simulink model "openloopresponse"  (R2018a)
settings: Solver=VariableStepAuto  StartTime=0.0  StopTime=130  RelTol=1e-3
values from neighbouring files (symbols this model uses):
  KT = 0.25    [DC_Motormfile.m]    (also in pid.m)
  L = 493*10^-9    (= 4.93e-07)    [DC_Motormfile.m]    (also in pid.m)
  R = 5.3*10^-3    (= 0.0053)    [DC_Motormfile.m]    (also in pid.m)
  Ts = 0.01    [pid.m]
libraries: simulink x2
settings Model: Creator=MAFAZ  LastModifiedBy=MAFAZ

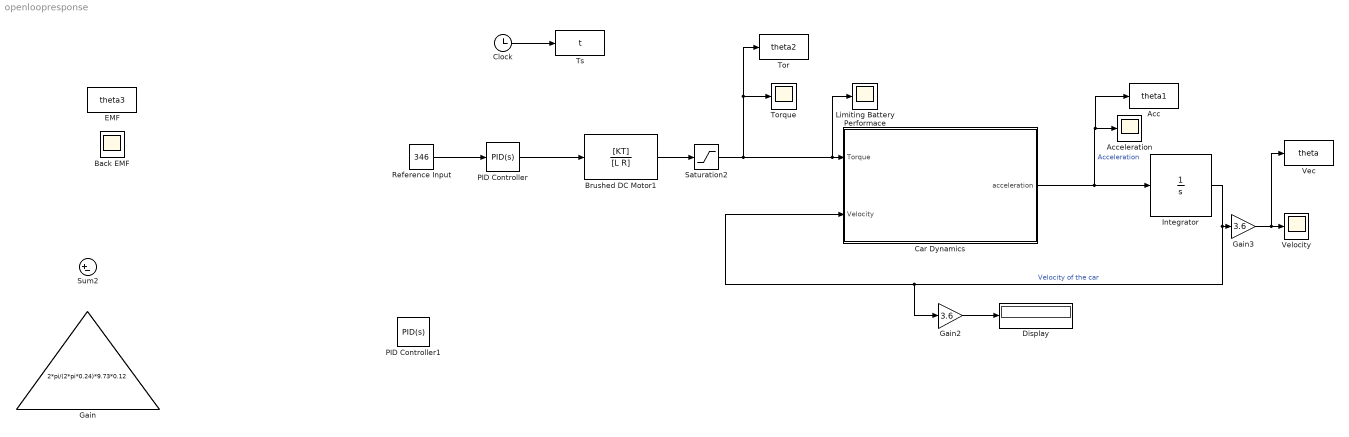
== system openloopresponse ==
  Acc : ToWorkspace  VariableName=theta1  SampleTime=Ts
  Acceleration : Scope
  Back EMF : Scope
  Brushed DC Motor1 : TransferFcn  Numerator=[KT]  Denominator=[L R]
  Car Dynamics : MATLAB Function  TreatAsAtomicUnit=on
  Clock : Clock
  Display : Display
  EMF : ToWorkspace  VariableName=theta3  SampleTime=Ts
  Gain : Gain  Gain=2*pi/(2*pi*0.24)*9.73*0.12
  Gain2 : Gain  Gain=3.6
  Gain3 : Gain  Gain=3.6
  Integrator : Integrator
  "Limiting Battery Performace " : Scope
  PID Controller : simulink/Continuous/PID Controller  Controller=PID  TimeDomain=Continuous-time  SampleTime=-1  IntegratorMethod=Forward Euler  FilterMethod=Forward Euler  Form=Parallel  UseFilter=on  ControllerParametersSource=internal  P=1000  I=500  D=0  N=100  InitialConditionSource=internal  InitialConditionForIntegrator=0  InitialConditionForFilter=0  ExternalReset=none  LimitOutput=on  UpperSaturationLimit=346  LowerSaturationLimit=0  LinearizeAsGain=on  AntiWindupMode=none  Kb=1  TrackingMode=off  Kt=1  PParamMin=[]  PParamMax=[]  IParamMin=[]  IParamMax=[]  DParamMin=[]  DParamMax=[]  NParamMin=[]  NParamMax=[]  KbParamMin=[]  KbParamMax=[]  KtParamMin=[]  KtParamMax=[]  POutMin=[]  POutMax=[]  IOutMin=[]  IOutMax=[]  DOutMin=[]  DOutMax=[]  NOutMin=[]  NOutMax=[]  KbOutMin=[]  KbOutMax=[]  KtOutMin=[]  KtOutMax=[]  IntegratorOutMin=[]  IntegratorOutMax=[]  FilterOutMin=[]  FilterOutMax=[]  SumOutMin=[]  SumOutMax=[]  SumI1OutMin=[]  SumI1OutMax=[]  SumI2OutMin=[]  SumI2OutMax=[]  SumI3OutMin=[]  SumI3OutMax=[]  SumDOutMin=[]  SumDOutMax=[]  SaturationOutMin=[]  SaturationOutMax=[]  IntegratorContinuousStateAttributes=''  IntegratorStateMustResolveToSignalObject=off  IntegratorRTWStateStorageClass=Auto  FilterContinuousStateAttributes=''  FilterStateMustResolveToSignalObject=off  FilterRTWStateStorageClass=Auto  DifferentiatorICPrevScaledInput=0  DifferentiatorOutMin=[]  DifferentiatorOutMax=[]  FilterDiffOutCoefMin=[]  FilterDiffOutCoefMax=[]  SumDenOutMin=[]  SumDenOutMax=[]  SumNumOutMin=[]  SumNumOutMax=[]  ReciprocalOutMin=[]  ReciprocalOutMax=[]  DivideOutMin=[]  DivideOutMax=[]  TunerSelectOption=Transfer Function Based (PID Tuner App)
  PID Controller1 : simulink/Continuous/PID Controller  Controller=PID  TimeDomain=Continuous-time  SampleTime=-1  IntegratorMethod=Forward Euler  FilterMethod=Forward Euler  Form=Parallel  UseFilter=on  ControllerParametersSource=internal  P=1  I=1  D=0  N=100  InitialConditionSource=internal  InitialConditionForIntegrator=0  InitialConditionForFilter=0  ExternalReset=none  LimitOutput=off  UpperSaturationLimit=inf  LowerSaturationLimit=-inf  LinearizeAsGain=on  AntiWindupMode=none  Kb=1  TrackingMode=off  Kt=1  PParamMin=[]  PParamMax=[]  IParamMin=[]  IParamMax=[]  DParamMin=[]  DParamMax=[]  NParamMin=[]  NParamMax=[]  KbParamMin=[]  KbParamMax=[]  KtParamMin=[]  KtParamMax=[]  POutMin=[]  POutMax=[]  IOutMin=[]  IOutMax=[]  DOutMin=[]  DOutMax=[]  NOutMin=[]  NOutMax=[]  KbOutMin=[]  KbOutMax=[]  KtOutMin=[]  KtOutMax=[]  IntegratorOutMin=[]  IntegratorOutMax=[]  FilterOutMin=[]  FilterOutMax=[]  SumOutMin=[]  SumOutMax=[]  SumI1OutMin=[]  SumI1OutMax=[]  SumI2OutMin=[]  SumI2OutMax=[]  SumI3OutMin=[]  SumI3OutMax=[]  SumDOutMin=[]  SumDOutMax=[]  SaturationOutMin=[]  SaturationOutMax=[]  IntegratorContinuousStateAttributes=''  IntegratorStateMustResolveToSignalObject=off  IntegratorRTWStateStorageClass=Auto  FilterContinuousStateAttributes=''  FilterStateMustResolveToSignalObject=off  FilterRTWStateStorageClass=Auto  DifferentiatorICPrevScaledInput=0  DifferentiatorOutMin=[]  DifferentiatorOutMax=[]  FilterDiffOutCoefMin=[]  FilterDiffOutCoefMax=[]  SumDenOutMin=[]  SumDenOutMax=[]  SumNumOutMin=[]  SumNumOutMax=[]  ReciprocalOutMin=[]  ReciprocalOutMax=[]  DivideOutMin=[]  DivideOutMax=[]  TunerSelectOption=Transfer Function Based (PID Tuner App)
  Reference Input : Constant  Value=346
  Saturation2 : Saturate  UpperLimit=600  LowerLimit=0
  Sum2 : Sum  Inputs=|+-
  Tor : ToWorkspace  VariableName=theta2  SampleTime=Ts
  "Torque " : Scope
  Ts : ToWorkspace  VariableName=t  SampleTime=Ts
  Vec : ToWorkspace  VariableName=theta  SampleTime=Ts
  Velocity : Scope
  wires:
  Car Dynamics/1(acceleration) -> Acc/1, Acceleration/1, Integrator/1  "Acceleration"
  Integrator/1 -> Gain3/1, Gain2/1, Car Dynamics/2(Velocity)  "Velocity of the car"
  Gain3/1 -> Vec/1, Velocity/1
  Reference Input/1 -> PID Controller/1
  Gain2/1 -> Display/1
  Brushed DC Motor1/1 -> Saturation2/1
  Clock/1 -> Ts/1
  Saturation2/1 -> "Limiting Battery Performace "/1, Car Dynamics/1(Torque), Tor/1, "Torque "/1
  PID Controller/1 -> Brushed DC Motor1/1

== matlab function openloopresponse/Car Dynamics ==
  data: Torque input; acceleration output; Velocity input
function acceleration = fcn(Torque, Velocity)
acceleration = (40.5*Torque*0.6-413-0.3381*Velocity^2)/2108;
